simulink subsystem "x6_dof_robot"  (R2023a)
settings: Solver=VariableStepAuto  StartTime=0.0  StopTime=10.0  RelTol=1e-3
undefined symbols (not defined in the file): forward_kinematics
settings Model: Creator=motya  LastModifiedBy=motya

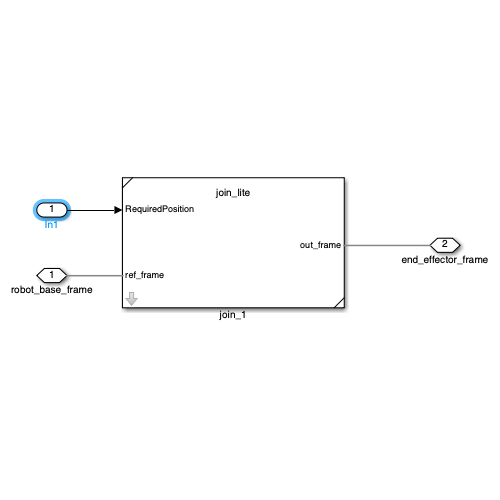
[thumbnail: Simulink's stored preview of the top-level diagram]
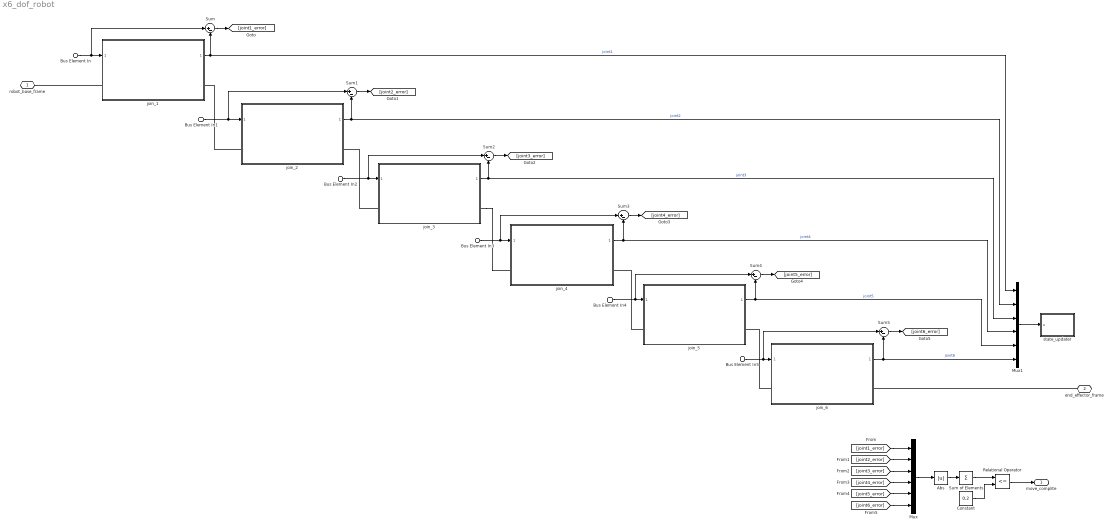
== system x6_dof_robot ==
  Bus Element In : Inport  PortName=setpoint  Element=joint1
  Bus Element In5 : Inport  PortName=setpoint  Element=joint6
  Bus Element In1 : Inport  PortName=setpoint  Element=joint2
  Bus Element In3 : Inport  PortName=setpoint  Element=joint4
  Bus Element In4 : Inport  PortName=setpoint  Element=joint5
  Bus Element In2 : Inport  PortName=setpoint  Element=joint3
  Abs : Abs  SaturateOnIntegerOverflow=off
  Constant : Constant  Value=0.2
  Mux : Mux  Inputs=6
  Mux1 : Mux  Inputs=6
  Relational Operator : RelationalOperator  Operator=<=  OutDataTypeStr=boolean  RndMeth=Simplest  InputSameDT=off
  Sum{,1..5} (6 alike) : Sum  Inputs=|+-
  Sum of Elements : Sum  Inputs=+
  join_1 : Subsystem  ReferencedSubsystem=join_lite  up_limit=180  low_limit=-180  out_frame_rot="forward_kinematics.zero_rot_between_frames(0,  0)"  out_frame_shift="forward_kinematics.zero_shift_between_frames(0,  0)"
  join_2 : Subsystem  ReferencedSubsystem=join_lite  up_limit=180  low_limit=-180  out_frame_rot="forward_kinematics.zero_rot_between_frames(0,  1)"  out_frame_shift="forward_kinematics.zero_shift_between_frames(0,  1)"
  join_3 : Subsystem  ReferencedSubsystem=join_lite  up_limit=180  low_limit=-180  out_frame_rot="forward_kinematics.zero_rot_between_frames(1,  2)"  out_frame_shift="forward_kinematics.zero_shift_between_frames(1,  2)"
  join_4 : Subsystem  ReferencedSubsystem=join_lite  up_limit=180  low_limit=-180  out_frame_rot="forward_kinematics.zero_rot_between_frames(2,  3)"  out_frame_shift="forward_kinematics.zero_shift_between_frames(2,  3)"
  join_5 : Subsystem  ReferencedSubsystem=join_lite  up_limit=180  low_limit=-180  out_frame_rot="forward_kinematics.zero_rot_between_frames(3,  4)"  out_frame_shift=forward_kinematics.zero_shift_between_frames(3, 4)
  join_6 : Subsystem  ReferencedSubsystem=join_lite  up_limit=180  low_limit=-180  out_frame_rot="forward_kinematics.zero_rot_between_frames(4,  5)"  out_frame_shift="forward_kinematics.zero_shift_between_frames(4,  5)"
  state_updater : MATLAB Function  TreatAsAtomicUnit=on
  robot_base_frame : PMIOPort  Side=Left
  end_effector_frame : PMIOPort  Port=2  Side=Right
  move_complite : Outport
  wires:
  Bus Element In/1 -> join_1/1, Sum/1
  Bus Element In1/1 -> join_2/1, Sum1/1
  Bus Element In2/1 -> join_3/1, Sum2/1
  Bus Element In3/1 -> join_4/1, Sum3/1
  Bus Element In4/1 -> join_5/1, Sum4/1
  Bus Element In5/1 -> join_6/1, Sum5/1
  join_1/1 -> Sum/2, Mux1/1  "joint1"
  join_2/1 -> Sum1/2, Mux1/2  "joint2"
  join_3/1 -> Sum2/2, Mux1/3  "joint3"
  join_4/1 -> Sum3/2, Mux1/4  "joint4"
  join_5/1 -> Sum4/2, Mux1/5  "joint5"
  join_6/1 -> Mux1/6, Sum5/2  "joint6"
  Mux1/1 -> state_updater/1(u)
  Sum/1 -> [joint1_error]
  Sum1/1 -> [joint2_error]
  Sum2/1 -> [joint3_error]
  Sum3/1 -> [joint4_error]
  Sum4/1 -> [joint5_error]
  Sum5/1 -> [joint6_error]
  Mux/1 -> Abs/1
  [joint1_error] -> Mux/1
  [joint2_error] -> Mux/2
  [joint3_error] -> Mux/3
  [joint4_error] -> Mux/4
  [joint5_error] -> Mux/5
  [joint6_error] -> Mux/6
  Abs/1 -> Sum of Elements/1
  Sum of Elements/1 -> Relational Operator/1
  Constant/1 -> Relational Operator/2
  Relational Operator/1 -> move_complite/1
  connections:
  join_1/LConn1 -- robot_base_frame/RConn1
  join_2/LConn1 -- join_1/RConn1
  join_3/LConn1 -- join_2/RConn1
  join_5/LConn1 -- join_4/RConn1
  join_3/RConn1 -- join_4/LConn1
  end_effector_frame/RConn1 -- join_6/RConn1
  join_6/LConn1 -- join_5/RConn1

== matlab function x6_dof_robot/state_updater ==
  data: u input
function fcn(u)
    inverse_kinematics.state_vector = u;
end
